simulink model "simple_kafka_producer_with_timestamp_example"  (R2020b)
settings: Solver=FixedStepAuto  StartTime=0.0  StopTime=inf  RelTol=1e-3
libraries: sl_kafka_lib x2
settings Model: EnablePacing=on  Creator=asolland  LastModifiedBy=asolland
settings DataIOCC: ReturnWorkspaceOutputs=off
settings OptimizationCC: DefaultParameterBehavior=Inlined  EnhancedBackFolding=on  PassReuseOutputArgsAs=Individual arguments  OptimizeBlockOrder=speed  DifferentSizesBufferReuse=on  OptimizationCustomize=off  EfficientTunableParamExpr=on
settings DebuggingCC: ParameterTunabilityLossMsg=error  ArithmeticOperatorsInVariantConditions=warning
settings HardwareCC: ProdBitPerLong=64  ProdLongLongMode=on  ProdHWDeviceType=Intel->x86-64 (Linux 64)
settings SFSimCC: MATLABDynamicMemAlloc=off  CustomCodeUndefinedFunction=UseInterfaceOnly
settings RTWCC: Description=Kafka Target  SystemTargetFile=kafkatarget.tlc  TemplateMakefile=ert_default_tmf  GenerateReport=on  RetainRTWFile=on  IncludeHyperlinkInReport=on  LaunchReport=on  GenerateTraceInfo=on  GenerateTraceReport=on  GenerateTraceReportSl=on  GenerateTraceReportSf=on  GenerateTraceReportEml=on
settings CodeAppCC: ForceParamTrailComments=on  IgnoreCustomStorageClasses=off  OperatorAnnotations=on  SimulinkDataObjDesc=on  SFDataObjDesc=on  InsertBlockDesc=on
settings STFCustomTargetCC: TargetLangStandard=C99 (ISO)  MultiwordLength=256  GenerateSampleERTMain=on  ConcurrentExecutionCompliant=off  CombineOutputUpdateFcns=on  ERTCustomFileBanners=on  SupportContinuousTime=off  SupportNonInlinedSFcns=off  RemoveResetFunc=on  MATLABClassNameForMDSCustomization=Simulink.SoftwareTarget.ERTCustomization  CPPClassGenCompliant=off  GRTInterface=off  UseToolchainInfoCompliant=on  SystemTargetFile=kafkatarget.tlc
settings ERTTargetCC: TargetLangStandard=C99 (ISO)  GenerateSampleERTMain=on  ParMdlRefBuildCompliant=off  CompOptLevelCompliant=off  ConcurrentExecutionCompliant=off  ModelStepFunctionPrototypeControlCompliant=off  CPPClassGenCompliant=off  InlinedParameterPlacement=NonHierarchical  ERTCustomFileTemplate=kafkatarget_process.tlc

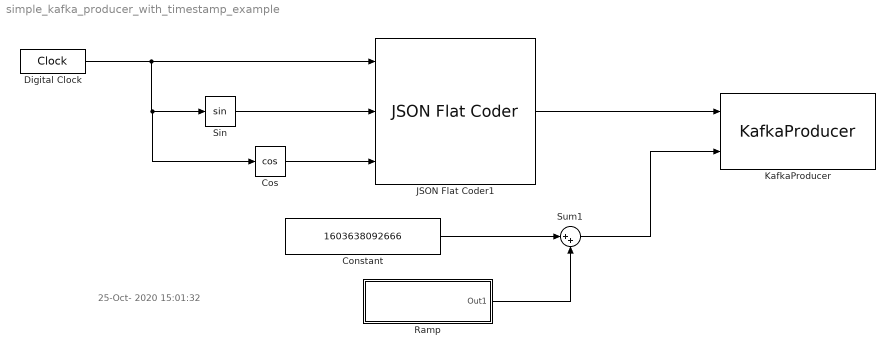
== system simple_kafka_producer_with_timestamp_example ==
  note: 25-Oct- 2020 15:01:32
  Constant : Constant  Value=1603638092666  OutDataTypeStr=int64
  Cos : Trigonometry  Operator=cos
  Digital Clock : DigitalClock
  JSON Flat Coder1 : sl_kafka_lib/JSON Flat Coder  sfpDirection=Encode  sfpLength=200  sfpFields={'X', 'Sine', 'Cosine'}  sfpOutLength=off  sfpInLength=on
  KafkaProducer : sl_kafka_lib/KafkaProducer  sfpBrokers='localhost:9092'  sfpTopic='testpub'  sfpKeyAsInput=off  sfpKeyAsInputLen=32  sfpKey='aKey'  sfpMsgLen=200  sfpTS=-1  sfpExtTimestamp=on  sfpConf=|  sfpTopicConf=compression.level=-1
      | client.id=sl_kafka_producer
      | message.copy.max.bytes=65535
  Ramp : Subsystem
  Sin : Trigonometry
  Sum1 : Sum  Inputs=|++
  wires:
  Constant/1 -> Sum1/1
  Cos/1 -> JSON Flat Coder1/3
  Sin/1 -> JSON Flat Coder1/2
  JSON Flat Coder1/1 -> KafkaProducer/1
  Digital Clock/1 -> Cos/1, Sin/1, JSON Flat Coder1/1
  Sum1/1 -> KafkaProducer/2
  Ramp/1(Out1) -> Sum1/2

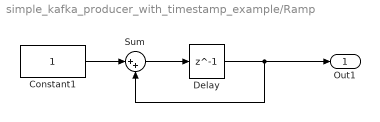
== system simple_kafka_producer_with_timestamp_example/Ramp ==
  Constant1 : Constant  OutDataTypeStr=int64
  Delay : Delay  DelayLength=1  SampleTime=1
  Sum : Sum  Inputs=|++
  Out1 : Outport
  wires:
  Constant1/1 -> Sum/1
  Delay/1 -> Out1/1, Sum/2
  Sum/1 -> Delay/1
